simulink model "IMU_Simulation_FxdPts"  (Simulink 7.9)
settings: Solver=FixedStepDiscrete  StartTime=0.0  StopTime=25  FixedStep=.001  RelTol=1e-3
PreLoadFcn:
  | Script_Kalman
values from neighbouring files (symbols this model uses):
  Az = [1 -Ts ;0 1]    [Script_Kalman.m]
  Kz = 1e-3*[.4 ; -.04]    [Script_Kalman.m]
  Ts = .001    (= 0.001)    [Script_Kalman.m]
undefined symbols (not defined in the file or in its folder): DiscIntNeverNeededParam
libraries: simulink x24
settings Model: Creator=Lubin  LastModifiedBy=denis.pretre
settings OptimizationCC: InitFltsAndDblsToZero=on
settings DebuggingCC: MultiTaskCondExecSysMsg=warning  MultiTaskRateTransMsg=warning  FcnCallInpInsideContextMsg=Use local settings  StrictBusMsg=Warning
settings HardwareCC: TargetHWDeviceType=32-bit Generic
settings GRTTargetCC: TargetFcnLib=ansi_tfl_tmw.mat  CombineOutputUpdateFcns=off  GRTInterface=on

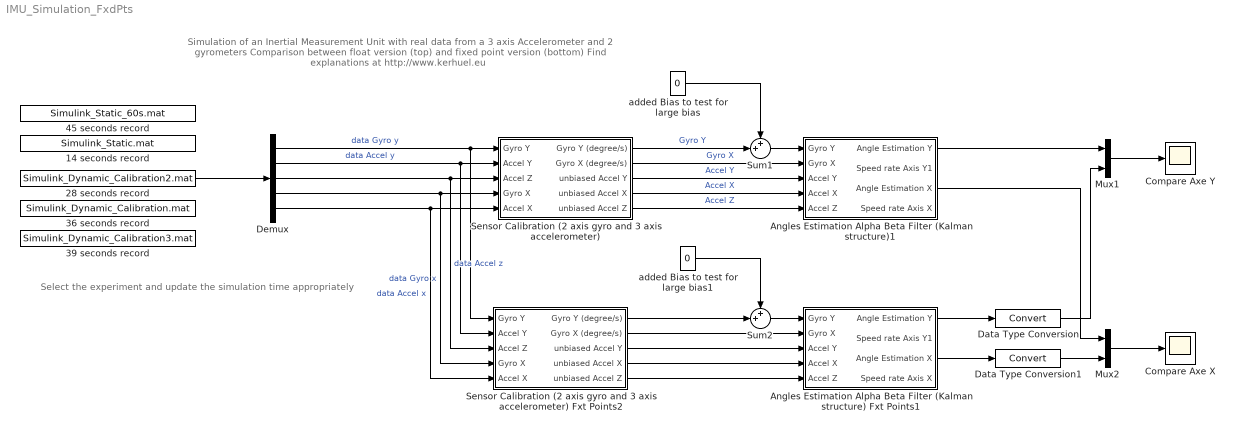
== system IMU_Simulation_FxdPts ==
  note: Simulation of an Inertial Measurement Unit with real data from a 3 axis Accelerometer and 2 gyrometers
      | Comparison between float version (top) and fixed point version (bottom)
      | Find explanations at http://www.kerhuel.eu
  note: Select the experiment and
      | update the simulation time appropriately
  14 seconds record : FromFile  FileName=Simulink_Static.mat  SampleTime=.001
  28 seconds record : FromFile  FileName=Simulink_Dynamic_Calibration2.mat  SampleTime=.001
  36 seconds record : FromFile  FileName=Simulink_Dynamic_Calibration.mat  SampleTime=.001
  39 seconds record : FromFile  FileName=Simulink_Dynamic_Calibration3.mat  SampleTime=.001
  45 seconds record : FromFile  FileName=Simulink_Static_60s.mat  SampleTime=.001
  Angles Estimation Alpha Beta Filter (Kalman structure) Fxt Points1 : Subsystem
  Angles Estimation Alpha Beta Filter (Kalman structure)1 : Subsystem
  Compare Axe X : Scope
      settings: TickLabels=on  TimeRange=25  YMin=-10  YMax=120  SaveName=ScopeData2  Decimation=10
  Compare Axe Y : Scope
      settings: TickLabels=on  TimeRange=25  YMin=0.4  YMax=1.25  SaveName=ScopeData4  Decimation=10
  Data Type Conversion : DataTypeConversion
  Data Type Conversion1 : DataTypeConversion
  Demux : Demux  Outputs=5
  Mux1 : Mux  Inputs=2
  Mux2 : Mux  Inputs=2
  Sensor Calibration (2 axis gyro and 3 axis accelerometer) : Subsystem
  Sensor Calibration (2 axis gyro and 3 axis accelerometer) Fxt Points2 : Subsystem
  Sum1 : Sum  Inputs=++|
  Sum2 : Sum  Inputs=++|
  added Bias to test for large bias : Constant  Value=0
  added Bias to test for large bias1 : Constant  Value=0  OutDataTypeStr=Inherit: Inherit via back propagation
  wires:
  Demux/2 -> Sensor Calibration (2 axis gyro and 3 axis accelerometer)/2(Accel Y), Sensor Calibration (2 axis gyro and 3 axis accelerometer) Fxt Points2/2(Accel Y)  "data Accel y"
  Demux/3 -> Sensor Calibration (2 axis gyro and 3 axis accelerometer)/3(Accel Z), Sensor Calibration (2 axis gyro and 3 axis accelerometer) Fxt Points2/3(Accel Z)  "data Accel z"
  Demux/4 -> Sensor Calibration (2 axis gyro and 3 axis accelerometer)/4(Gyro X), Sensor Calibration (2 axis gyro and 3 axis accelerometer) Fxt Points2/4(Gyro X)  "data Gyro x"
  Demux/5 -> Sensor Calibration (2 axis gyro and 3 axis accelerometer)/5(Accel X), Sensor Calibration (2 axis gyro and 3 axis accelerometer) Fxt Points2/5(Accel X)  "data Accel x"
  Demux/1 -> Sensor Calibration (2 axis gyro and 3 axis accelerometer)/1(Gyro Y), Sensor Calibration (2 axis gyro and 3 axis accelerometer) Fxt Points2/1(Gyro Y)  "data Gyro y"
  Sensor Calibration (2 axis gyro and 3 axis accelerometer)/1(Gyro Y (degree/s)) -> Sum1/2  "Gyro Y"
  Sensor Calibration (2 axis gyro and 3 axis accelerometer)/2(Gyro X (degree/s)) -> Angles Estimation Alpha Beta Filter (Kalman structure)1/2(Gyro X)  "Gyro X"
  Sensor Calibration (2 axis gyro and 3 axis accelerometer)/3(unbiased Accel Y) -> Angles Estimation Alpha Beta Filter (Kalman structure)1/3(Accel Y)  "Accel Y"
  Sensor Calibration (2 axis gyro and 3 axis accelerometer)/4(unbiased Accel X) -> Angles Estimation Alpha Beta Filter (Kalman structure)1/4(Accel X)  "Accel X"
  Sensor Calibration (2 axis gyro and 3 axis accelerometer)/5(unbiased Accel Z) -> Angles Estimation Alpha Beta Filter (Kalman structure)1/5(Accel Z)  "Accel Z"
  Sum1/1 -> Angles Estimation Alpha Beta Filter (Kalman structure)1/1(Gyro Y)
  Mux1/1 -> Compare Axe Y/1
  Sensor Calibration (2 axis gyro and 3 axis accelerometer) Fxt Points2/2(Gyro X (degree/s)) -> Angles Estimation Alpha Beta Filter (Kalman structure) Fxt Points1/2(Gyro X)
  Sensor Calibration (2 axis gyro and 3 axis accelerometer) Fxt Points2/4(unbiased Accel X) -> Angles Estimation Alpha Beta Filter (Kalman structure) Fxt Points1/4(Accel X)
  Sensor Calibration (2 axis gyro and 3 axis accelerometer) Fxt Points2/5(unbiased Accel Z) -> Angles Estimation Alpha Beta Filter (Kalman structure) Fxt Points1/5(Accel Z)
  Angles Estimation Alpha Beta Filter (Kalman structure)1/1(Angle Estimation Y) -> Mux1/1
  Angles Estimation Alpha Beta Filter (Kalman structure) Fxt Points1/1(Angle Estimation Y) -> Data Type Conversion/1
  Data Type Conversion/1 -> Mux1/2
  added Bias to test for large bias/1 -> Sum1/1
  Mux2/1 -> Compare Axe X/1
  Angles Estimation Alpha Beta Filter (Kalman structure) Fxt Points1/3(Angle Estimation X) -> Data Type Conversion1/1
  Data Type Conversion1/1 -> Mux2/2
  Angles Estimation Alpha Beta Filter (Kalman structure)1/3(Angle Estimation X) -> Mux2/1
  Sensor Calibration (2 axis gyro and 3 axis accelerometer) Fxt Points2/3(unbiased Accel Y) -> Angles Estimation Alpha Beta Filter (Kalman structure) Fxt Points1/3(Accel Y)
  28 seconds record/1 -> Demux/1
  added Bias to test for large bias1/1 -> Sum2/1
  Sensor Calibration (2 axis gyro and 3 axis accelerometer) Fxt Points2/1(Gyro Y (degree/s)) -> Sum2/2
  Sum2/1 -> Angles Estimation Alpha Beta Filter (Kalman structure) Fxt Points1/1(Gyro Y)

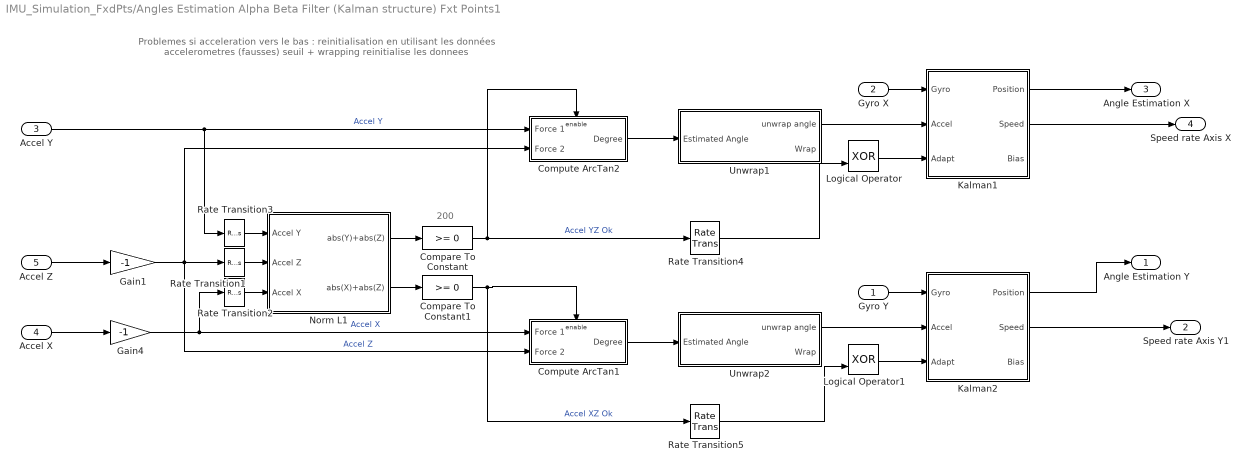
== system IMU_Simulation_FxdPts/Angles Estimation Alpha Beta Filter (Kalman structure) Fxt Points1 ==
  note: 200
  note: Problemes si acceleration vers le bas : reinitialisation en utilisant les données accelerometres (fausses)
      | seuil + wrapping reinitialise les donnees
  Gyro Y : Inport
  Gyro X : Inport  Port=2
  Accel Y : Inport  Port=3
  Accel X : Inport  Port=4
  Accel Z : Inport  Port=5
  Compare To Constant : simulink/Logic and Bit Operations/Compare To Constant  relop=>=  const=0  OutDataTypeStr=boolean  ZeroCross=off
  Compare To Constant1 : simulink/Logic and Bit Operations/Compare To Constant  relop=>=  const=0  OutDataTypeStr=boolean  ZeroCross=off
  Compute ArcTan1 : Subsystem
  Compute ArcTan2 : Subsystem
  Gain1 : Gain  Gain=-1  OutDataTypeStr=Inherit: Same as input
  Gain4 : Gain  Gain=-1  OutDataTypeStr=Inherit: Same as input
  Kalman1 : Subsystem
  Kalman2 : Subsystem
  Logical Operator : Logic  Operator=XOR  AllPortsSameDT=off  OutDataTypeStr=boolean
  Logical Operator1 : Logic  Operator=XOR  AllPortsSameDT=off  OutDataTypeStr=boolean
  Norm L1 : Subsystem
  Rate Transition1 : RateTransition  Integrity=off  OutPortSampleTime=.2
  Rate Transition2 : RateTransition  Integrity=off  OutPortSampleTime=.2
  Rate Transition3 : RateTransition  Integrity=off  OutPortSampleTime=.2
  Rate Transition4 : RateTransition  Integrity=off  OutPortSampleTime=.001
  Rate Transition5 : RateTransition  Integrity=off  OutPortSampleTime=.001
  Unwrap1 : Subsystem
  Unwrap2 : Subsystem
  Angle Estimation Y : Outport
  Speed rate Axis Y1 : Outport  Port=2
  Angle Estimation X : Outport  Port=3
  Speed rate Axis X : Outport  Port=4
  wires:
  Kalman2/2(Speed) -> Speed rate Axis Y1/1
  Kalman1/2(Speed) -> Speed rate Axis X/1
  Unwrap2/1(unwrap angle) -> Kalman2/2(Accel)
  Logical Operator/1 -> Kalman1/3(Adapt)
  Rate Transition5/1 -> Logical Operator1/2
  Gain1/1 -> Compute ArcTan1/2(Force 2), Compute ArcTan2/2(Force 2), Rate Transition1/1  "Accel Z"
  Logical Operator1/1 -> Kalman2/3(Adapt)
  Rate Transition4/1 -> Logical Operator/2
  Unwrap1/1(unwrap angle) -> Kalman1/2(Accel)
  Rate Transition3/1 -> Norm L1/1(Accel Y)
  Rate Transition2/1 -> Norm L1/3(Accel X)
  Rate Transition1/1 -> Norm L1/2(Accel Z)
  Kalman2/1(Position) -> Angle Estimation Y/1
  Kalman1/1(Position) -> Angle Estimation X/1
  Compare To Constant1/1 -> Compute ArcTan1/Enable, Rate Transition5/1  "Accel XZ Ok"
  Compare To Constant/1 -> Compute ArcTan2/Enable, Rate Transition4/1  "Accel YZ Ok"
  Norm L1/1(abs(Y)+abs(Z)) -> Compare To Constant/1
  Norm L1/2(abs(X)+abs(Z)) -> Compare To Constant1/1
  Accel Z/1 -> Gain1/1
  Gain4/1 -> Compute ArcTan1/1(Force 1), Rate Transition2/1  "Accel X"
  Compute ArcTan2/1(Degree) -> Unwrap1/1(Estimated Angle)
  Compute ArcTan1/1(Degree) -> Unwrap2/1(Estimated Angle)
  Accel X/1 -> Gain4/1
  Accel Y/1 -> Rate Transition3/1, Compute ArcTan2/1(Force 1)  "Accel Y"
  Gyro X/1 -> Kalman1/1(Gyro)
  Gyro Y/1 -> Kalman2/1(Gyro)

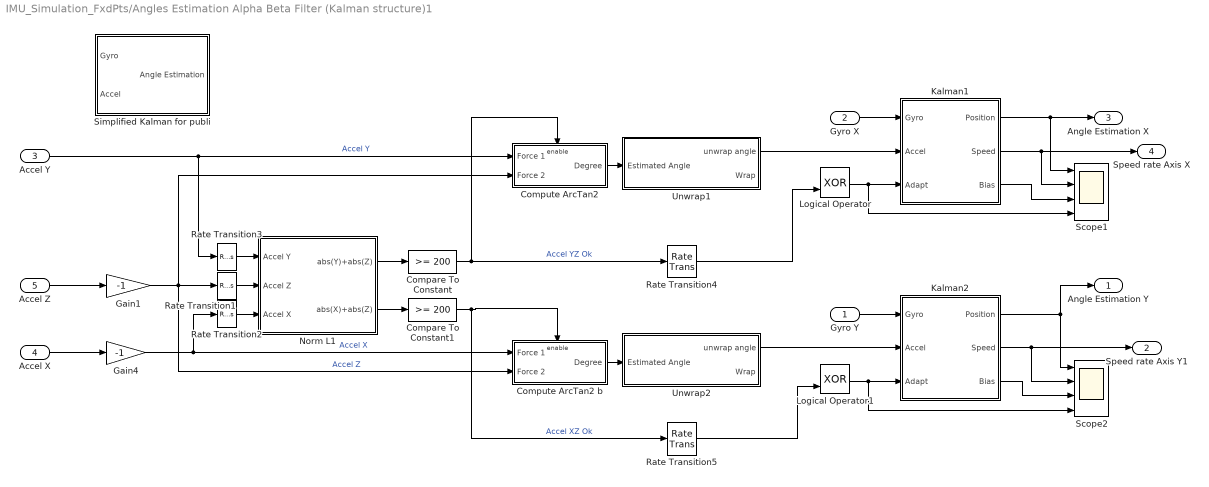
== system IMU_Simulation_FxdPts/Angles Estimation Alpha Beta Filter (Kalman structure)1 ==
  Gyro Y : Inport
  Gyro X : Inport  Port=2
  Accel Y : Inport  Port=3
  Accel X : Inport  Port=4
  Accel Z : Inport  Port=5
  Compare To Constant : simulink/Logic and Bit Operations/Compare To Constant  relop=>=  const=200  OutDataTypeStr=boolean  ZeroCross=off
  Compare To Constant1 : simulink/Logic and Bit Operations/Compare To Constant  relop=>=  const=200  OutDataTypeStr=boolean  ZeroCross=off
  Compute ArcTan2 : Subsystem
  Compute ArcTan2 b : Subsystem
  Gain1 : Gain  Gain=-1
  Gain4 : Gain  Gain=-1
  Kalman1 : Subsystem
  Kalman2 : Subsystem
  Logical Operator : Logic  Operator=XOR  AllPortsSameDT=off  OutDataTypeStr=boolean
  Logical Operator1 : Logic  Operator=XOR  AllPortsSameDT=off  OutDataTypeStr=boolean
  Norm L1 : Subsystem
  Rate Transition1 : RateTransition  Integrity=off  OutPortSampleTime=.2
  Rate Transition2 : RateTransition  Integrity=off  OutPortSampleTime=.2
  Rate Transition3 : RateTransition  Integrity=off  OutPortSampleTime=.2
  Rate Transition4 : RateTransition  Integrity=off  OutPortSampleTime=.001
  Rate Transition5 : RateTransition  Integrity=off  OutPortSampleTime=.001
  Scope1 : Scope  NumInputPorts=4
      settings: TimeRange=9.424342105263159  YMin=-375~-20~-27.5~0  YMax=-150~40~2.5~1
  Scope2 : Scope  NumInputPorts=4
      settings: TimeRange=9.424342105263159  YMin=-375~-20~-27.5~0  YMax=-150~40~2.5~1
  Simplified Kalman for publi : Subsystem
  Unwrap1 : Subsystem
  Unwrap2 : Subsystem
  Angle Estimation Y : Outport
  Speed rate Axis Y1 : Outport  Port=2
  Angle Estimation X : Outport  Port=3
  Speed rate Axis X : Outport  Port=4
  wires:
  Kalman1/3(Bias) -> Scope1/3
  Kalman2/3(Bias) -> Scope2/3
  Kalman2/2(Speed) -> Speed rate Axis Y1/1, Scope2/2
  Kalman1/2(Speed) -> Speed rate Axis X/1, Scope1/2
  Unwrap2/1(unwrap angle) -> Kalman2/2(Accel)
  Logical Operator/1 -> Scope1/4, Kalman1/3(Adapt)
  Rate Transition5/1 -> Logical Operator1/2
  Gain1/1 -> Rate Transition1/1, Compute ArcTan2/2(Force 2), Compute ArcTan2 b/2(Force 2)  "Accel Z"
  Logical Operator1/1 -> Kalman2/3(Adapt), Scope2/4
  Rate Transition4/1 -> Logical Operator/2
  Unwrap1/1(unwrap angle) -> Kalman1/2(Accel)
  Rate Transition3/1 -> Norm L1/1(Accel Y)
  Rate Transition2/1 -> Norm L1/3(Accel X)
  Rate Transition1/1 -> Norm L1/2(Accel Z)
  Kalman2/1(Position) -> Scope2/1, Angle Estimation Y/1
  Kalman1/1(Position) -> Scope1/1, Angle Estimation X/1
  Compare To Constant1/1 -> Rate Transition5/1, Compute ArcTan2 b/Enable  "Accel XZ Ok"
  Compare To Constant/1 -> Rate Transition4/1, Compute ArcTan2/Enable  "Accel YZ Ok"
  Norm L1/1(abs(Y)+abs(Z)) -> Compare To Constant/1
  Norm L1/2(abs(X)+abs(Z)) -> Compare To Constant1/1
  Accel Z/1 -> Gain1/1
  Gain4/1 -> Rate Transition2/1, Compute ArcTan2 b/1(Force 1)  "Accel X"
  Compute ArcTan2/1(Degree) -> Unwrap1/1(Estimated Angle)
  Compute ArcTan2 b/1(Degree) -> Unwrap2/1(Estimated Angle)
  Accel X/1 -> Gain4/1
  Accel Y/1 -> Compute ArcTan2/1(Force 1), Rate Transition3/1  "Accel Y"
  Gyro X/1 -> Kalman1/1(Gyro)
  Gyro Y/1 -> Kalman2/1(Gyro)

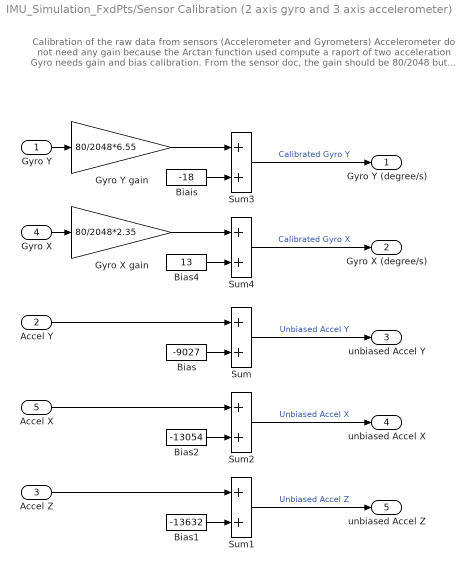
== system IMU_Simulation_FxdPts/Sensor Calibration (2 axis gyro and 3 axis accelerometer) ==
  note: Calibration of the raw data from sensors (Accelerometer and Gyrometers)
      | Accelerometer do not need any gain because the Arctan function used compute a raport of two acceleration
      | Gyro needs gain and bias calibration. From the sensor doc, the gain should be 80/2048 but...
  Gyro Y : Inport
  Accel Y : Inport  Port=2
  Accel Z : Inport  Port=3
  Gyro X : Inport  Port=4
  Accel X : Inport  Port=5
  "Biais " : Constant  Value=-18
  Bias : Constant  Value=-9027
  Bias1 : Constant  Value=-13632
  Bias2 : Constant  Value=-13054
  Bias4 : Constant  Value=13
  Gyro X gain : Gain  Gain=80/2048*2.35  OutDataTypeStr=float('double')
  Gyro Y gain : Gain  Gain=80/2048*6.55  OutDataTypeStr=float('double')
  Sum{,1..4} (5 alike) : Sum
  Gyro Y (degree/s) : Outport
  Gyro X (degree/s) : Outport  Port=2
  unbiased Accel Y : Outport  Port=3
  unbiased Accel X : Outport  Port=4
  unbiased Accel Z : Outport  Port=5
  wires:
  Bias/1 -> Sum/2
  Bias1/1 -> Sum1/2
  Bias2/1 -> Sum2/2
  Gyro Y/1 -> Gyro Y gain/1
  Accel Y/1 -> Sum/1
  Sum/1 -> unbiased Accel Y/1  "Unbiased Accel Y"
  Accel Z/1 -> Sum1/1
  Sum1/1 -> unbiased Accel Z/1  "Unbiased Accel Z"
  Gyro X/1 -> Gyro X gain/1
  Accel X/1 -> Sum2/1
  Sum2/1 -> unbiased Accel X/1  "Unbiased Accel X"
  Gyro Y gain/1 -> Sum3/1
  Sum3/1 -> Gyro Y (degree/s)/1  "Calibrated Gyro Y"
  "Biais "/1 -> Sum3/2
  Gyro X gain/1 -> Sum4/1
  Sum4/1 -> Gyro X (degree/s)/1  "Calibrated Gyro X"
  Bias4/1 -> Sum4/2

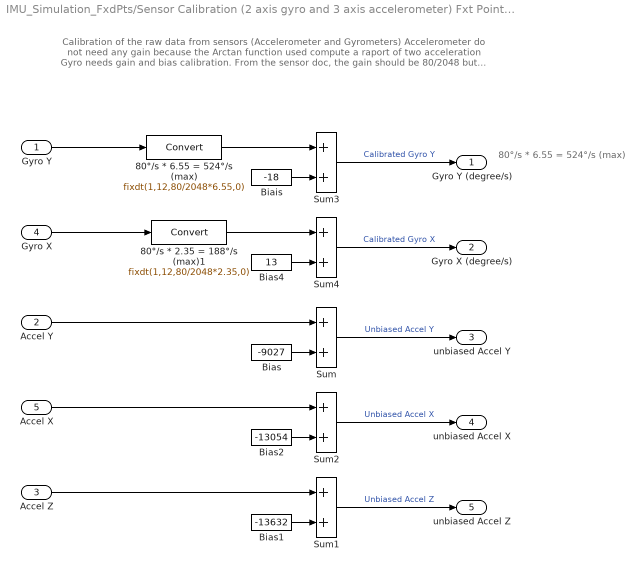
== system IMU_Simulation_FxdPts/Sensor Calibration (2 axis gyro and 3 axis accelerometer) Fxt Points2 ==
  note: Calibration of the raw data from sensors (Accelerometer and Gyrometers)
      | Accelerometer do not need any gain because the Arctan function used compute a raport of two acceleration
      | Gyro needs gain and bias calibration. From the sensor doc, the gain should be 80/2048 but...
  note: 80°/s * 6.55 = 524°/s (max)
  Gyro Y : Inport
  Accel Y : Inport  Port=2
  Accel Z : Inport  Port=3
  Gyro X : Inport  Port=4
  Accel X : Inport  Port=5
  80°/s * 2.35 = 188°/s (max)1 : DataTypeConversion  OutDataTypeStr=fixdt(1,12,80/2048*2.35,0)  ConvertRealWorld=Stored Integer (SI)
  80°/s * 6.55 = 524°/s (max) : DataTypeConversion  OutDataTypeStr=fixdt(1,12,80/2048*6.55,0)  ConvertRealWorld=Stored Integer (SI)
  "Biais " : Constant  Value=-18  OutDataTypeStr=Inherit: Inherit via back propagation
  Bias : Constant  Value=-9027  OutDataTypeStr=Inherit: Inherit via back propagation
  Bias1 : Constant  Value=-13632  OutDataTypeStr=Inherit: Inherit via back propagation
  Bias2 : Constant  Value=-13054  OutDataTypeStr=Inherit: Inherit via back propagation
  Bias4 : Constant  Value=13  OutDataTypeStr=Inherit: Inherit via back propagation
  Sum : Sum  OutDataTypeStr=int16
  Sum1 : Sum  OutDataTypeStr=int16
  Sum2 : Sum  OutDataTypeStr=int16
  Sum3 : Sum
  Sum4 : Sum
  Gyro Y (degree/s) : Outport
  Gyro X (degree/s) : Outport  Port=2
  unbiased Accel Y : Outport  Port=3
  unbiased Accel X : Outport  Port=4
  unbiased Accel Z : Outport  Port=5
  wires:
  Bias4/1 -> Sum4/2
  Sum4/1 -> Gyro X (degree/s)/1  "Calibrated Gyro X"
  80°/s * 2.35 = 188°/s (max)1/1 -> Sum4/1
  "Biais "/1 -> Sum3/2
  Sum3/1 -> Gyro Y (degree/s)/1  "Calibrated Gyro Y"
  80°/s * 6.55 = 524°/s (max)/1 -> Sum3/1
  Sum2/1 -> unbiased Accel X/1  "Unbiased Accel X"
  Accel X/1 -> Sum2/1
  Gyro X/1 -> 80°/s * 2.35 = 188°/s (max)1/1
  Sum1/1 -> unbiased Accel Z/1  "Unbiased Accel Z"
  Accel Z/1 -> Sum1/1
  Sum/1 -> unbiased Accel Y/1  "Unbiased Accel Y"
  Accel Y/1 -> Sum/1
  Gyro Y/1 -> 80°/s * 6.55 = 524°/s (max)/1
  Bias2/1 -> Sum2/2
  Bias1/1 -> Sum1/2
  Bias/1 -> Sum/2

== system IMU_Simulation_FxdPts/Angles Estimation Alpha Beta Filter (Kalman structure) Fxt Points1/Compute ArcTan1 ==
  Force 1 : Inport
  Force 2 : Inport  Port=2
  Enable : EnablePort  StatesWhenEnabling=reset
  180/pi : DataTypeConversion  OutDataTypeStr=fixdt(1,16,180/pi*2^-12,0)  ConvertRealWorld=Stored Integer (SI)
  80°/s * 6.55 = 524°/s (max) : DataTypeConversion  OutDataTypeStr=single
  80°/s * 6.55 = 524°/s (max)1 : DataTypeConversion  OutDataTypeStr=single
  80°/s * 6.55 = 524°/s (max)2 : DataTypeConversion  OutDataTypeStr=fixdt(1,16,12)
  Trigonometric Function1 : Trigonometry  Operator=atan2  OutputSignalType=real
  Degree : Outport
  wires:
  Trigonometric Function1/1 -> 80°/s * 6.55 = 524°/s (max)2/1
  180/pi/1 -> Degree/1
  Force 1/1 -> 80°/s * 6.55 = 524°/s (max)/1
  Force 2/1 -> 80°/s * 6.55 = 524°/s (max)1/1
  80°/s * 6.55 = 524°/s (max)/1 -> Trigonometric Function1/1
  80°/s * 6.55 = 524°/s (max)1/1 -> Trigonometric Function1/2
  80°/s * 6.55 = 524°/s (max)2/1 -> 180/pi/1

== system IMU_Simulation_FxdPts/Angles Estimation Alpha Beta Filter (Kalman structure) Fxt Points1/Compute ArcTan2 ==
  Force 1 : Inport
  Force 2 : Inport  Port=2
  Enable : EnablePort  StatesWhenEnabling=reset
  180/pi : DataTypeConversion  OutDataTypeStr=fixdt(1,16,180/pi*2^-12,0)  ConvertRealWorld=Stored Integer (SI)
  80°/s * 6.55 = 524°/s (max) : DataTypeConversion  OutDataTypeStr=single
  80°/s * 6.55 = 524°/s (max)1 : DataTypeConversion  OutDataTypeStr=single
  80°/s * 6.55 = 524°/s (max)2 : DataTypeConversion  OutDataTypeStr=fixdt(1,16,12)
  Trigonometric Function1 : Trigonometry  Operator=atan2  OutputSignalType=real
  Degree : Outport
  wires:
  80°/s * 6.55 = 524°/s (max)2/1 -> 180/pi/1
  80°/s * 6.55 = 524°/s (max)1/1 -> Trigonometric Function1/2
  80°/s * 6.55 = 524°/s (max)/1 -> Trigonometric Function1/1
  Force 2/1 -> 80°/s * 6.55 = 524°/s (max)1/1
  Force 1/1 -> 80°/s * 6.55 = 524°/s (max)/1
  180/pi/1 -> Degree/1
  Trigonometric Function1/1 -> 80°/s * 6.55 = 524°/s (max)2/1

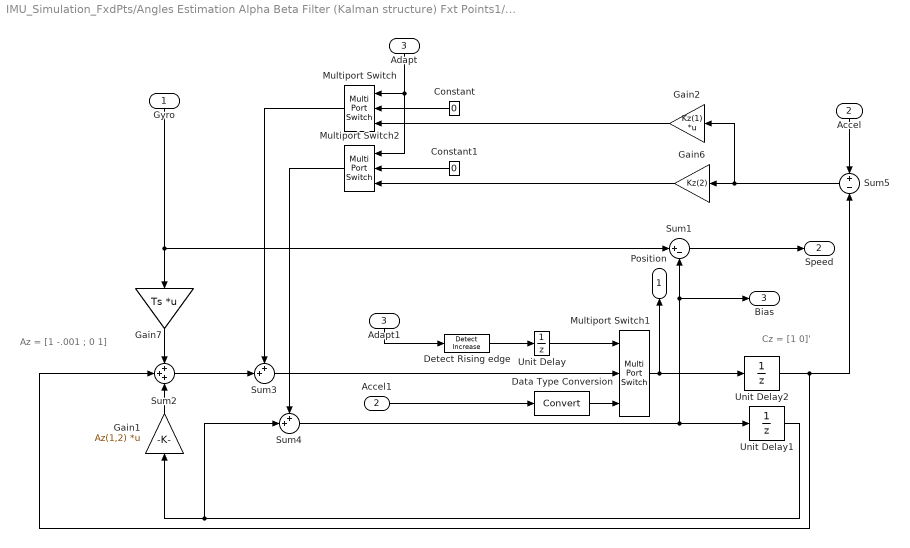
== system IMU_Simulation_FxdPts/Angles Estimation Alpha Beta Filter (Kalman structure) Fxt Points1/Kalman1 ==
  note: Az = [1 -.001 ; 0 1]
  note: Cz = [1 0]'
  Gyro : Inport
  Accel : Inport  Port=2
  Adapt : Inport  Port=3
  Accel1 : InportShadow  Port=2
  Adapt1 : InportShadow  Port=3
  Constant : Constant  Value=0  OutDataTypeStr=Inherit: Inherit via back propagation
  Constant1 : Constant  Value=0  OutDataTypeStr=Inherit: Inherit via back propagation
  Data Type Conversion : DataTypeConversion
  Detect Rising edge : simulink/Logic and Bit Operations/Detect Increase  vinit=0  InputProcessing=Inherited  OutDataTypeStr=uint8
  Gain1 : Gain  Gain=Az(1,2)  Multiplication=Matrix(K*u)  OutDataTypeStr=fixdt(1,32,36)
  Gain2 : Gain  Gain=Kz(1)  Multiplication=Matrix(K*u)  ParamDataTypeStr=fixdt(1,32,42)  OutDataTypeStr=fixdt(1,16,20)  SaturateOnIntegerOverflow=on
  Gain6 : Gain  Gain=Kz(2)  ParamDataTypeStr=fixdt(1,32,45)  OutDataTypeStr=fixdt(1,16,23)  SaturateOnIntegerOverflow=on
  Gain7 : Gain  Gain=Ts  Multiplication=Matrix(K*u)  OutDataTypeStr=Inherit: Inherit via back propagation
  Multiport Switch : MultiPortSwitch  DataPortOrder=Zero-based contiguous  Inputs=2  zeroidx=on
  Multiport Switch1 : MultiPortSwitch  DataPortOrder=Zero-based contiguous  Inputs=2  zeroidx=on  OutDataTypeStr=Inherit: Inherit via back propagation
  Multiport Switch2 : MultiPortSwitch  DataPortOrder=Zero-based contiguous  Inputs=2  zeroidx=on
  Sum1 : Sum  Inputs=|+-  OutDataTypeStr=Inherit: Same as first input
  Sum2 : Sum  Inputs=+++  OutDataTypeStr=fixdt(1,32,22)
  Sum3 : Sum  Inputs=++|  OutDataTypeStr=fixdt(1,32,22)
  Sum4 : Sum  Inputs=++|  OutDataTypeStr=fixdt(1,32,26)
  Sum5 : Sum  Inputs=+-  OutDataTypeStr=fixdt(1,16,9)  SaturateOnIntegerOverflow=on
  Unit Delay : UnitDelay  SampleTime=-1
  Unit Delay1 : UnitDelay  SampleTime=-1
  Unit Delay2 : UnitDelay  SampleTime=-1
  Position : Outport  OutDataTypeStr=fixdt(1,32,22)
  Speed : Outport  Port=2
  Bias : Outport  Port=3
  wires:
  Gyro/1 -> Sum1/1, Gain7/1
  Gain6/1 -> Multiport Switch2/3
  Unit Delay1/1 -> Sum4/2, Gain1/1
  Multiport Switch1/1 -> Position/1, Unit Delay2/1
  Sum4/1 -> Bias/1, Sum1/2, Unit Delay1/1
  Data Type Conversion/1 -> Multiport Switch1/3
  Accel1/1 -> Data Type Conversion/1
  Sum3/1 -> Multiport Switch1/2
  Multiport Switch2/1 -> Sum4/1
  Multiport Switch/1 -> Sum3/1
  Constant1/1 -> Multiport Switch2/2
  Gain2/1 -> Multiport Switch/3
  Gain1/1 -> Sum2/3
  Sum1/1 -> Speed/1
  Unit Delay/1 -> Multiport Switch1/1
  Accel/1 -> Sum5/1
  Gain7/1 -> Sum2/1
  Sum5/1 -> Gain2/1, Gain6/1
  Sum2/1 -> Sum3/2
  Unit Delay2/1 -> Sum2/2, Sum5/2
  Adapt/1 -> Multiport Switch2/1, Multiport Switch/1
  Constant/1 -> Multiport Switch/2
  Detect Rising edge/1 -> Unit Delay/1
  Adapt1/1 -> Detect Rising edge/1

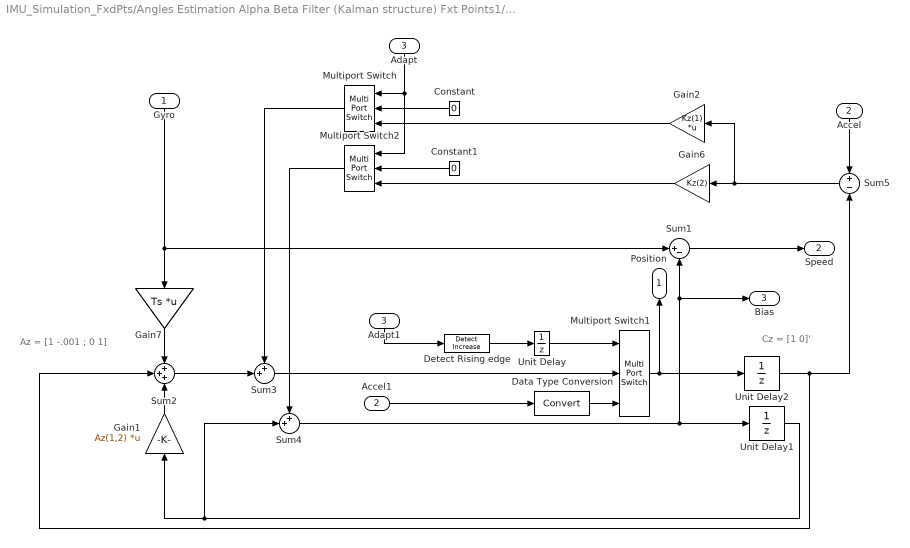
== system IMU_Simulation_FxdPts/Angles Estimation Alpha Beta Filter (Kalman structure) Fxt Points1/Kalman2 ==
  note: Cz = [1 0]'
  note: Az = [1 -.001 ; 0 1]
  Gyro : Inport
  Accel : Inport  Port=2
  Adapt : Inport  Port=3
  Accel1 : InportShadow  Port=2
  Adapt1 : InportShadow  Port=3
  Constant : Constant  Value=0  OutDataTypeStr=Inherit: Inherit via back propagation
  Constant1 : Constant  Value=0  OutDataTypeStr=Inherit: Inherit via back propagation
  Data Type Conversion : DataTypeConversion
  Detect Rising edge : simulink/Logic and Bit Operations/Detect Increase  vinit=0  InputProcessing=Inherited  OutDataTypeStr=uint8
  Gain1 : Gain  Gain=Az(1,2)  Multiplication=Matrix(K*u)  OutDataTypeStr=fixdt(1,32,36)
  Gain2 : Gain  Gain=Kz(1)  Multiplication=Matrix(K*u)  ParamDataTypeStr=fixdt(1,32,42)  OutDataTypeStr=fixdt(1,16,20)  SaturateOnIntegerOverflow=on
  Gain6 : Gain  Gain=Kz(2)  ParamDataTypeStr=fixdt(1,32,45)  OutDataTypeStr=fixdt(1,16,23)  SaturateOnIntegerOverflow=on
  Gain7 : Gain  Gain=Ts  Multiplication=Matrix(K*u)  OutDataTypeStr=Inherit: Inherit via back propagation
  Multiport Switch : MultiPortSwitch  DataPortOrder=Zero-based contiguous  Inputs=2  zeroidx=on
  Multiport Switch1 : MultiPortSwitch  DataPortOrder=Zero-based contiguous  Inputs=2  zeroidx=on  OutDataTypeStr=Inherit: Inherit via back propagation
  Multiport Switch2 : MultiPortSwitch  DataPortOrder=Zero-based contiguous  Inputs=2  zeroidx=on
  Sum1 : Sum  Inputs=|+-  OutDataTypeStr=Inherit: Same as first input
  Sum2 : Sum  Inputs=+++  OutDataTypeStr=fixdt(1,32,22)
  Sum3 : Sum  Inputs=++|  OutDataTypeStr=fixdt(1,32,22)
  Sum4 : Sum  Inputs=++|  OutDataTypeStr=fixdt(1,32,26)
  Sum5 : Sum  Inputs=+-  OutDataTypeStr=fixdt(1,16,9)  SaturateOnIntegerOverflow=on
  Unit Delay : UnitDelay  SampleTime=-1
  Unit Delay1 : UnitDelay  SampleTime=-1
  Unit Delay2 : UnitDelay  SampleTime=-1
  Position : Outport  OutDataTypeStr=fixdt(1,32,22)
  Speed : Outport  Port=2
  Bias : Outport  Port=3
  wires:
  Adapt1/1 -> Detect Rising edge/1
  Detect Rising edge/1 -> Unit Delay/1
  Constant/1 -> Multiport Switch/2
  Adapt/1 -> Multiport Switch/1, Multiport Switch2/1
  Unit Delay2/1 -> Sum5/2, Sum2/2
  Sum2/1 -> Sum3/2
  Sum5/1 -> Gain6/1, Gain2/1
  Gain7/1 -> Sum2/1
  Accel/1 -> Sum5/1
  Unit Delay/1 -> Multiport Switch1/1
  Sum1/1 -> Speed/1
  Gain1/1 -> Sum2/3
  Gain2/1 -> Multiport Switch/3
  Constant1/1 -> Multiport Switch2/2
  Multiport Switch/1 -> Sum3/1
  Multiport Switch2/1 -> Sum4/1
  Sum3/1 -> Multiport Switch1/2
  Accel1/1 -> Data Type Conversion/1
  Data Type Conversion/1 -> Multiport Switch1/3
  Sum4/1 -> Unit Delay1/1, Sum1/2, Bias/1
  Multiport Switch1/1 -> Unit Delay2/1, Position/1
  Unit Delay1/1 -> Gain1/1, Sum4/2
  Gain6/1 -> Multiport Switch2/3
  Gyro/1 -> Gain7/1, Sum1/1

== system IMU_Simulation_FxdPts/Angles Estimation Alpha Beta Filter (Kalman structure) Fxt Points1/Norm L1 ==
  Accel Y : Inport
  Accel Z : Inport  Port=2
  Accel X : Inport  Port=3
  Abs : Abs
  Abs1 : Abs
  Abs2 : Abs
  Sum1 : Sum
  Sum3 : Sum
  abs(Y)+abs(Z) : Outport
  abs(X)+abs(Z) : Outport  Port=2
  wires:
  Sum1/1 -> abs(X)+abs(Z)/1
  Accel X/1 -> Abs2/1
  Abs2/1 -> Sum1/2
  Sum3/1 -> abs(Y)+abs(Z)/1
  Accel Z/1 -> Abs1/1
  Accel Y/1 -> Abs/1
  Abs1/1 -> Sum3/2, Sum1/1
  Abs/1 -> Sum3/1

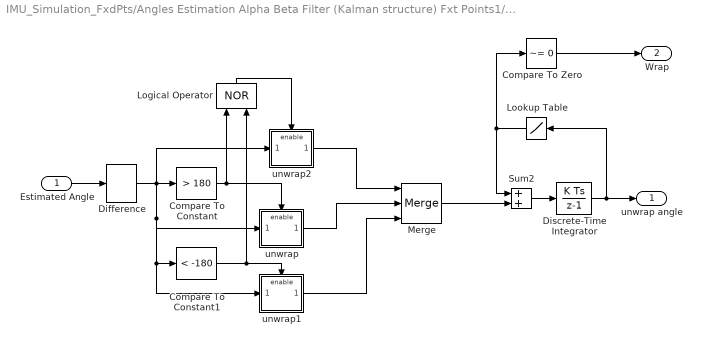
== system IMU_Simulation_FxdPts/Angles Estimation Alpha Beta Filter (Kalman structure) Fxt Points1/Unwrap1 ==
  Estimated Angle : Inport
  Compare To Constant : simulink/Logic and Bit Operations/Compare To Constant  relop=>  const=180  OutDataTypeStr=uint8  ZeroCross=off
  Compare To Constant1 : simulink/Logic and Bit Operations/Compare To Constant  relop=<  const=-180  OutDataTypeStr=uint8  ZeroCross=off
  Compare To Zero : simulink/Logic and Bit Operations/Compare To Zero  relop=~=  OutDataTypeStr=uint8  ZeroCross=off
  Difference : simulink/Discrete/Difference  ICPrevInput=0.0  InputProcessing=Inherited  OutMin=[]  OutMax=[]  OutDataType=sfix(16)  OutScaling=2^-10  DoSatur=off
  Discrete-Time Integrator : DiscreteIntegrator  gainval=1000  SampleTime=-1  ICPrevOutput=DiscIntNeverNeededParam  ICPrevScaledInput=DiscIntNeverNeededParam
  Logical Operator : Logic  Operator=NOR  AllPortsSameDT=off  OutDataTypeStr=boolean
  Lookup Table : Lookup  InputValues=[-450 -195 195]  Table=[+360 0 -360]  LookUpMeth=Use Input Below
  Merge : Merge  Inputs=3
  Sum2 : Sum
  unwrap : Subsystem  TreatAsAtomicUnit=on
  unwrap1 : Subsystem  TreatAsAtomicUnit=on
  unwrap2 : Subsystem  TreatAsAtomicUnit=on
  unwrap angle : Outport
  Wrap : Outport  Port=2
  wires:
  Discrete-Time Integrator/1 -> unwrap angle/1, Lookup Table/1
  Estimated Angle/1 -> Difference/1
  unwrap1/1(Out1) -> Merge/3
  unwrap/1(Out1) -> Merge/2
  unwrap2/1(Out1) -> Merge/1
  Logical Operator/1 -> unwrap2/Enable
  Compare To Constant1/1 -> Logical Operator/2, unwrap1/Enable
  Compare To Constant/1 -> unwrap/Enable, Logical Operator/1
  Difference/1 -> unwrap2/1(In1), unwrap1/1(In1), Compare To Constant1/1, unwrap/1(In1), Compare To Constant/1
  Sum2/1 -> Discrete-Time Integrator/1
  Merge/1 -> Sum2/2
  Lookup Table/1 -> Sum2/1, Compare To Zero/1
  Compare To Zero/1 -> Wrap/1

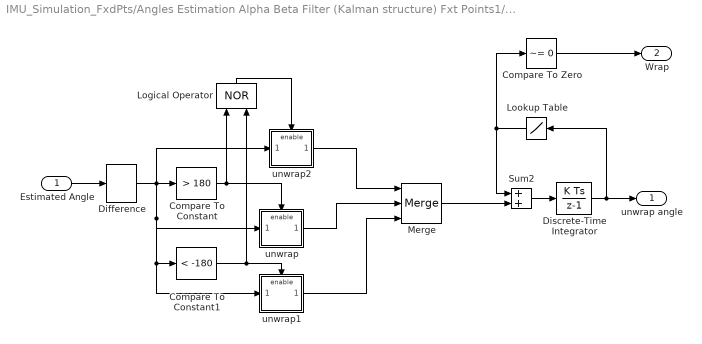
== system IMU_Simulation_FxdPts/Angles Estimation Alpha Beta Filter (Kalman structure) Fxt Points1/Unwrap2 ==
  Estimated Angle : Inport
  Compare To Constant : simulink/Logic and Bit Operations/Compare To Constant  relop=>  const=180  OutDataTypeStr=uint8  ZeroCross=off
  Compare To Constant1 : simulink/Logic and Bit Operations/Compare To Constant  relop=<  const=-180  OutDataTypeStr=uint8  ZeroCross=off
  Compare To Zero : simulink/Logic and Bit Operations/Compare To Zero  relop=~=  OutDataTypeStr=uint8  ZeroCross=off
  Difference : simulink/Discrete/Difference  ICPrevInput=0.0  InputProcessing=Inherited  OutMin=[]  OutMax=[]  OutDataType=sfix(16)  OutScaling=2^-10  DoSatur=off
  Discrete-Time Integrator : DiscreteIntegrator  gainval=1000  SampleTime=-1  ICPrevOutput=DiscIntNeverNeededParam  ICPrevScaledInput=DiscIntNeverNeededParam
  Logical Operator : Logic  Operator=NOR  AllPortsSameDT=off  OutDataTypeStr=boolean
  Lookup Table : Lookup  InputValues=[-450 -195 195]  Table=[+360 0 -360]  LookUpMeth=Use Input Below
  Merge : Merge  Inputs=3
  Sum2 : Sum
  unwrap : Subsystem  TreatAsAtomicUnit=on
  unwrap1 : Subsystem  TreatAsAtomicUnit=on
  unwrap2 : Subsystem  TreatAsAtomicUnit=on
  unwrap angle : Outport
  Wrap : Outport  Port=2
  wires:
  Compare To Zero/1 -> Wrap/1
  Lookup Table/1 -> Compare To Zero/1, Sum2/1
  Merge/1 -> Sum2/2
  Sum2/1 -> Discrete-Time Integrator/1
  Difference/1 -> Compare To Constant/1, unwrap/1(In1), Compare To Constant1/1, unwrap1/1(In1), unwrap2/1(In1)
  Compare To Constant/1 -> Logical Operator/1, unwrap/Enable
  Compare To Constant1/1 -> unwrap1/Enable, Logical Operator/2
  Logical Operator/1 -> unwrap2/Enable
  unwrap2/1(Out1) -> Merge/1
  unwrap/1(Out1) -> Merge/2
  unwrap1/1(Out1) -> Merge/3
  Estimated Angle/1 -> Difference/1
  Discrete-Time Integrator/1 -> Lookup Table/1, unwrap angle/1

== system IMU_Simulation_FxdPts/Angles Estimation Alpha Beta Filter (Kalman structure)1/Compute ArcTan2 ==
  Force 1 : Inport
  Force 2 : Inport  Port=2
  Enable : EnablePort  StatesWhenEnabling=reset
  Gain1 : Gain  Gain=180/pi  OutDataTypeStr=float('double')
  Trigonometric Function1 : Trigonometry  Operator=atan2  OutputSignalType=real
  Degree : Outport
  wires:
  Force 2/1 -> Trigonometric Function1/2
  Force 1/1 -> Trigonometric Function1/1
  Gain1/1 -> Degree/1
  Trigonometric Function1/1 -> Gain1/1

== system IMU_Simulation_FxdPts/Angles Estimation Alpha Beta Filter (Kalman structure)1/Compute ArcTan2 b ==
  Force 1 : Inport
  Force 2 : Inport  Port=2
  Enable : EnablePort  StatesWhenEnabling=reset
  Gain1 : Gain  Gain=180/pi  OutDataTypeStr=float('double')
  Trigonometric Function1 : Trigonometry  Operator=atan2  OutputSignalType=real
  Degree : Outport
  wires:
  Trigonometric Function1/1 -> Gain1/1
  Gain1/1 -> Degree/1
  Force 1/1 -> Trigonometric Function1/1
  Force 2/1 -> Trigonometric Function1/2

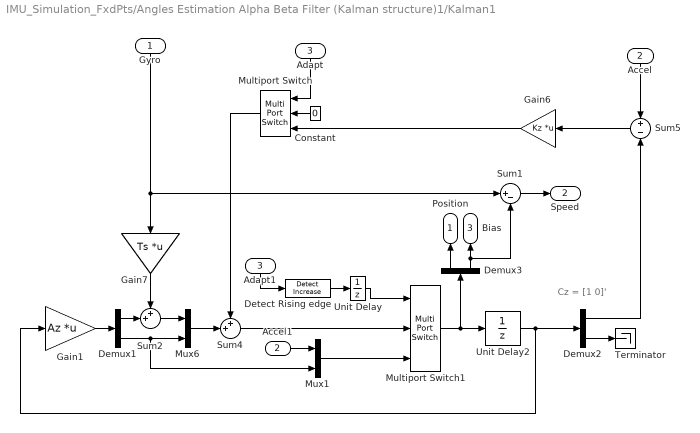
== system IMU_Simulation_FxdPts/Angles Estimation Alpha Beta Filter (Kalman structure)1/Kalman1 ==
  note: Cz = [1 0]'
  Gyro : Inport
  Accel : Inport  Port=2
  Adapt : Inport  Port=3
  Accel1 : InportShadow  Port=2
  Adapt1 : InportShadow  Port=3
  Constant : Constant  Value=0
  Demux1 : Demux  Outputs=2
  Demux2 : Demux  Outputs=2
  Demux3 : Demux  Outputs=2
  Detect Rising edge : simulink/Logic and Bit Operations/Detect Increase  vinit=0  InputProcessing=Inherited  OutDataTypeStr=uint8
  Gain1 : Gain  Gain=Az  Multiplication=Matrix(K*u)
  Gain6 : Gain  Gain=Kz  Multiplication=Matrix(K*u)
  Gain7 : Gain  Gain=Ts  Multiplication=Matrix(K*u)
  Multiport Switch : MultiPortSwitch  DataPortOrder=Zero-based contiguous  Inputs=2  zeroidx=on
  Multiport Switch1 : MultiPortSwitch  DataPortOrder=Zero-based contiguous  Inputs=2  zeroidx=on
  Mux1 : Mux  Inputs=2
  Mux6 : Mux  Inputs=2
  Sum1 : Sum  Inputs=|+-
  Sum2 : Sum  Inputs=++|
  Sum4 : Sum  Inputs=++|
  Sum5 : Sum  Inputs=+-
  Terminator : Terminator
  Unit Delay : UnitDelay  SampleTime=-1
  Unit Delay2 : UnitDelay  SampleTime=-1
  Position : Outport
  Speed : Outport  Port=2
  Bias : Outport  Port=3
  wires:
  Demux2/2 -> Terminator/1
  Mux1/1 -> Multiport Switch1/3
  Accel1/1 -> Mux1/1
  Adapt1/1 -> Detect Rising edge/1
  Sum4/1 -> Multiport Switch1/2
  Multiport Switch1/1 -> Unit Delay2/1, Demux3/1
  Detect Rising edge/1 -> Unit Delay/1
  Constant/1 -> Multiport Switch/2
  Gain6/1 -> Multiport Switch/3
  Adapt/1 -> Multiport Switch/1
  Multiport Switch/1 -> Sum4/1
  Demux2/1 -> Sum5/2
  Gain1/1 -> Demux1/1
  Demux1/1 -> Sum2/2
  Sum2/1 -> Mux6/1
  Demux1/2 -> Mux1/2, Mux6/2
  Mux6/1 -> Sum4/2
  Sum5/1 -> Gain6/1
  Gain7/1 -> Sum2/1
  Accel/1 -> Sum5/1
  Gyro/1 -> Gain7/1, Sum1/1
  Unit Delay/1 -> Multiport Switch1/1
  Unit Delay2/1 -> Demux2/1, Gain1/1
  Demux3/1 -> Position/1
  Demux3/2 -> Bias/1, Sum1/2
  Sum1/1 -> Speed/1

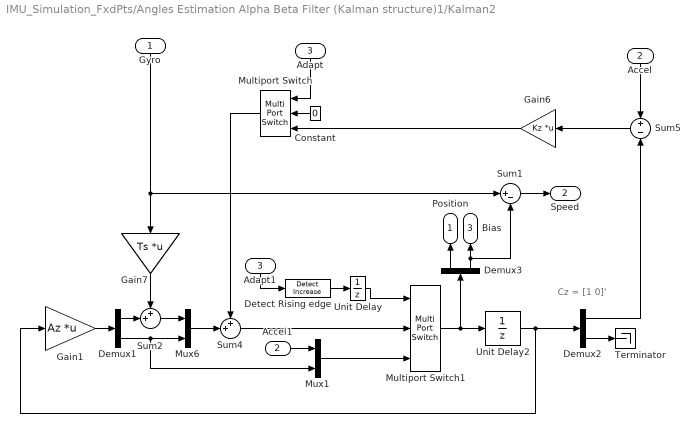
== system IMU_Simulation_FxdPts/Angles Estimation Alpha Beta Filter (Kalman structure)1/Kalman2 ==
  note: Cz = [1 0]'
  Gyro : Inport
  Accel : Inport  Port=2
  Adapt : Inport  Port=3
  Accel1 : InportShadow  Port=2
  Adapt1 : InportShadow  Port=3
  Constant : Constant  Value=0
  Demux1 : Demux  Outputs=2
  Demux2 : Demux  Outputs=2
  Demux3 : Demux  Outputs=2
  Detect Rising edge : simulink/Logic and Bit Operations/Detect Increase  vinit=0  InputProcessing=Inherited  OutDataTypeStr=uint8
  Gain1 : Gain  Gain=Az  Multiplication=Matrix(K*u)
  Gain6 : Gain  Gain=Kz  Multiplication=Matrix(K*u)
  Gain7 : Gain  Gain=Ts  Multiplication=Matrix(K*u)
  Multiport Switch : MultiPortSwitch  DataPortOrder=Zero-based contiguous  Inputs=2  zeroidx=on
  Multiport Switch1 : MultiPortSwitch  DataPortOrder=Zero-based contiguous  Inputs=2  zeroidx=on
  Mux1 : Mux  Inputs=2
  Mux6 : Mux  Inputs=2
  Sum1 : Sum  Inputs=|+-
  Sum2 : Sum  Inputs=++|
  Sum4 : Sum  Inputs=++|  OutDataTypeStr=Inherit: Inherit via back propagation
  Sum5 : Sum  Inputs=+-
  Terminator : Terminator
  Unit Delay : UnitDelay  SampleTime=-1
  Unit Delay2 : UnitDelay  SampleTime=-1
  Position : Outport
  Speed : Outport  Port=2
  Bias : Outport  Port=3
  wires:
  Sum1/1 -> Speed/1
  Demux3/2 -> Sum1/2, Bias/1
  Demux3/1 -> Position/1
  Unit Delay2/1 -> Gain1/1, Demux2/1
  Unit Delay/1 -> Multiport Switch1/1
  Gyro/1 -> Sum1/1, Gain7/1
  Accel/1 -> Sum5/1
  Gain7/1 -> Sum2/1
  Sum5/1 -> Gain6/1
  Mux6/1 -> Sum4/2
  Demux1/2 -> Mux6/2, Mux1/2
  Sum2/1 -> Mux6/1
  Demux1/1 -> Sum2/2
  Gain1/1 -> Demux1/1
  Demux2/1 -> Sum5/2
  Multiport Switch/1 -> Sum4/1
  Adapt/1 -> Multiport Switch/1
  Gain6/1 -> Multiport Switch/3
  Constant/1 -> Multiport Switch/2
  Detect Rising edge/1 -> Unit Delay/1
  Multiport Switch1/1 -> Demux3/1, Unit Delay2/1
  Sum4/1 -> Multiport Switch1/2
  Adapt1/1 -> Detect Rising edge/1
  Accel1/1 -> Mux1/1
  Mux1/1 -> Multiport Switch1/3
  Demux2/2 -> Terminator/1

== system IMU_Simulation_FxdPts/Angles Estimation Alpha Beta Filter (Kalman structure)1/Norm L1 ==
  Accel Y : Inport
  Accel Z : Inport  Port=2
  Accel X : Inport  Port=3
  Abs : Abs
  Abs1 : Abs
  Abs2 : Abs
  Sum1 : Sum
  Sum3 : Sum
  abs(Y)+abs(Z) : Outport
  abs(X)+abs(Z) : Outport  Port=2
  wires:
  Sum1/1 -> abs(X)+abs(Z)/1
  Accel X/1 -> Abs2/1
  Abs2/1 -> Sum1/2
  Sum3/1 -> abs(Y)+abs(Z)/1
  Accel Z/1 -> Abs1/1
  Accel Y/1 -> Abs/1
  Abs1/1 -> Sum3/2, Sum1/1
  Abs/1 -> Sum3/1

== system IMU_Simulation_FxdPts/Angles Estimation Alpha Beta Filter (Kalman structure)1/Simplified Kalman for publi ==
  note: Cz = [1 0]'
  Gyro : Inport
  Accel : Inport  Port=2
  Demux1 : Demux  Outputs=2
  Demux2 : Demux  Outputs=2
  Gain1 : Gain  Gain=Az  Multiplication=Matrix(K*u)
  Gain6 : Gain  Gain=Kz  Multiplication=Matrix(K*u)
  Gain7 : Gain  Gain=Ts  Multiplication=Matrix(K*u)
  Mux6 : Mux  Inputs=2
  Sum2 : Sum  Inputs=++|
  Sum4 : Sum  Inputs=++|
  Sum5 : Sum  Inputs=+-
  Terminator : Terminator
  Unit Delay2 : UnitDelay  SampleTime=-1
  Angle Estimation : Outport
  wires:
  Gain6/1 -> Sum4/1
  Unit Delay2/1 -> Gain1/1, Demux2/1
  Gyro/1 -> Gain7/1
  Accel/1 -> Sum5/1
  Gain7/1 -> Sum2/1
  Sum5/1 -> Gain6/1
  Mux6/1 -> Sum4/2
  Demux1/2 -> Mux6/2  "Gyro Bias"
  Sum2/1 -> Mux6/1  "Angle Estimation"
  Demux1/1 -> Sum2/2
  Gain1/1 -> Demux1/1
  Demux2/1 -> Angle Estimation/1, Sum5/2
  Sum4/1 -> Unit Delay2/1
  Demux2/2 -> Terminator/1

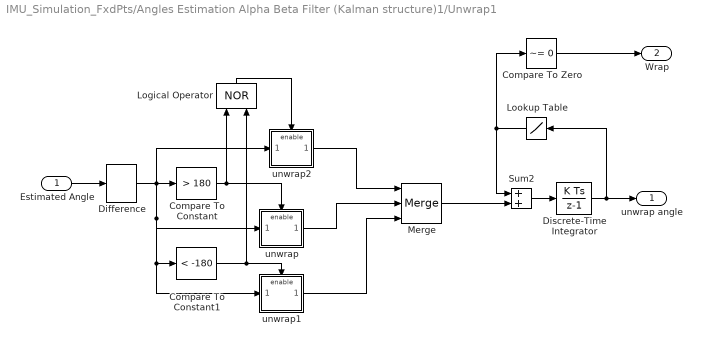
== system IMU_Simulation_FxdPts/Angles Estimation Alpha Beta Filter (Kalman structure)1/Unwrap1 ==
  Estimated Angle : Inport
  Compare To Constant : simulink/Logic and Bit Operations/Compare To Constant  relop=>  const=180  OutDataTypeStr=uint8  ZeroCross=off
  Compare To Constant1 : simulink/Logic and Bit Operations/Compare To Constant  relop=<  const=-180  OutDataTypeStr=uint8  ZeroCross=off
  Compare To Zero : simulink/Logic and Bit Operations/Compare To Zero  relop=~=  OutDataTypeStr=uint8  ZeroCross=off
  Difference : simulink/Discrete/Difference  ICPrevInput=0.0  InputProcessing=Inherited  OutMin=[]  OutMax=[]  OutDataType=sfix(16)  OutScaling=2^-10  DoSatur=off
  Discrete-Time Integrator : DiscreteIntegrator  gainval=1000  SampleTime=-1  ICPrevOutput=DiscIntNeverNeededParam  ICPrevScaledInput=DiscIntNeverNeededParam
  Logical Operator : Logic  Operator=NOR  AllPortsSameDT=off  OutDataTypeStr=boolean
  Lookup Table : Lookup  InputValues=[-500 -195 195]  Table=[+360 0 -360]  LookUpMeth=Use Input Below
  Merge : Merge  Inputs=3
  Sum2 : Sum
  unwrap : Subsystem  TreatAsAtomicUnit=on
  unwrap1 : Subsystem  TreatAsAtomicUnit=on
  unwrap2 : Subsystem  TreatAsAtomicUnit=on
  unwrap angle : Outport
  Wrap : Outport  Port=2
  wires:
  Discrete-Time Integrator/1 -> unwrap angle/1, Lookup Table/1
  Estimated Angle/1 -> Difference/1
  unwrap1/1(Out1) -> Merge/3
  unwrap/1(Out1) -> Merge/2
  unwrap2/1(Out1) -> Merge/1
  Logical Operator/1 -> unwrap2/Enable
  Compare To Constant1/1 -> Logical Operator/2, unwrap1/Enable
  Compare To Constant/1 -> unwrap/Enable, Logical Operator/1
  Difference/1 -> unwrap2/1(In1), unwrap1/1(In1), Compare To Constant1/1, unwrap/1(In1), Compare To Constant/1
  Sum2/1 -> Discrete-Time Integrator/1
  Merge/1 -> Sum2/2
  Lookup Table/1 -> Sum2/1, Compare To Zero/1
  Compare To Zero/1 -> Wrap/1

== system IMU_Simulation_FxdPts/Angles Estimation Alpha Beta Filter (Kalman structure)1/Unwrap2 ==
  Estimated Angle : Inport
  Compare To Constant : simulink/Logic and Bit Operations/Compare To Constant  relop=>  const=180  OutDataTypeStr=uint8  ZeroCross=off
  Compare To Constant1 : simulink/Logic and Bit Operations/Compare To Constant  relop=<  const=-180  OutDataTypeStr=uint8  ZeroCross=off
  Compare To Zero : simulink/Logic and Bit Operations/Compare To Zero  relop=~=  OutDataTypeStr=uint8  ZeroCross=off
  Difference : simulink/Discrete/Difference  ICPrevInput=0.0  InputProcessing=Inherited  OutMin=[]  OutMax=[]  OutDataType=sfix(16)  OutScaling=2^-10  DoSatur=off
  Discrete-Time Integrator : DiscreteIntegrator  gainval=1000  SampleTime=-1  ICPrevOutput=DiscIntNeverNeededParam  ICPrevScaledInput=DiscIntNeverNeededParam
  Logical Operator : Logic  Operator=NOR  AllPortsSameDT=off  OutDataTypeStr=boolean
  Lookup Table : Lookup  InputValues=[-500 -195 195]  Table=[+360 0 -360]  LookUpMeth=Use Input Below
  Merge : Merge  Inputs=3
  Sum2 : Sum
  unwrap : Subsystem  TreatAsAtomicUnit=on
  unwrap1 : Subsystem  TreatAsAtomicUnit=on
  unwrap2 : Subsystem  TreatAsAtomicUnit=on
  unwrap angle : Outport
  Wrap : Outport  Port=2
  wires:
  Compare To Zero/1 -> Wrap/1
  Lookup Table/1 -> Compare To Zero/1, Sum2/1
  Merge/1 -> Sum2/2
  Sum2/1 -> Discrete-Time Integrator/1
  Difference/1 -> Compare To Constant/1, unwrap/1(In1), Compare To Constant1/1, unwrap1/1(In1), unwrap2/1(In1)
  Compare To Constant/1 -> Logical Operator/1, unwrap/Enable
  Compare To Constant1/1 -> unwrap1/Enable, Logical Operator/2
  Logical Operator/1 -> unwrap2/Enable
  unwrap2/1(Out1) -> Merge/1
  unwrap/1(Out1) -> Merge/2
  unwrap1/1(Out1) -> Merge/3
  Estimated Angle/1 -> Difference/1
  Discrete-Time Integrator/1 -> Lookup Table/1, unwrap angle/1

== system IMU_Simulation_FxdPts/Angles Estimation Alpha Beta Filter (Kalman structure) Fxt Points1/Unwrap1/unwrap ==
  In1 : Inport
  Enable : EnablePort
  Bias2 : Constant  Value=-360  OutDataTypeStr=Inherit: Inherit via back propagation
  Sum2 : Sum  OutDataTypeStr=Inherit: Same as first input
  Out1 : Outport
  wires:
  Bias2/1 -> Sum2/2
  Sum2/1 -> Out1/1
  In1/1 -> Sum2/1

== system IMU_Simulation_FxdPts/Angles Estimation Alpha Beta Filter (Kalman structure) Fxt Points1/Unwrap1/unwrap1 ==
  In1 : Inport
  Enable : EnablePort
  Bias2 : Constant  Value=360  OutDataTypeStr=Inherit: Inherit via back propagation
  Sum2 : Sum  OutDataTypeStr=Inherit: Same as first input
  Out1 : Outport
  wires:
  Sum2/1 -> Out1/1
  Bias2/1 -> Sum2/2
  In1/1 -> Sum2/1

== system IMU_Simulation_FxdPts/Angles Estimation Alpha Beta Filter (Kalman structure) Fxt Points1/Unwrap1/unwrap2 ==
  In1 : Inport
  Enable : EnablePort
  Out1 : Outport
  wires:
  In1/1 -> Out1/1

== system IMU_Simulation_FxdPts/Angles Estimation Alpha Beta Filter (Kalman structure) Fxt Points1/Unwrap2/unwrap ==
  In1 : Inport
  Enable : EnablePort
  Bias2 : Constant  Value=-360  OutDataTypeStr=Inherit: Inherit via back propagation
  Sum2 : Sum  OutDataTypeStr=Inherit: Same as first input
  Out1 : Outport
  wires:
  In1/1 -> Sum2/1
  Sum2/1 -> Out1/1
  Bias2/1 -> Sum2/2

== system IMU_Simulation_FxdPts/Angles Estimation Alpha Beta Filter (Kalman structure) Fxt Points1/Unwrap2/unwrap1 ==
  In1 : Inport
  Enable : EnablePort
  Bias2 : Constant  Value=360  OutDataTypeStr=Inherit: Inherit via back propagation
  Sum2 : Sum  OutDataTypeStr=Inherit: Same as first input
  Out1 : Outport
  wires:
  In1/1 -> Sum2/1
  Bias2/1 -> Sum2/2
  Sum2/1 -> Out1/1

== system IMU_Simulation_FxdPts/Angles Estimation Alpha Beta Filter (Kalman structure) Fxt Points1/Unwrap2/unwrap2 ==
  In1 : Inport
  Enable : EnablePort
  Out1 : Outport
  wires:
  In1/1 -> Out1/1

== system IMU_Simulation_FxdPts/Angles Estimation Alpha Beta Filter (Kalman structure)1/Unwrap1/unwrap ==
  In1 : Inport
  Enable : EnablePort
  Bias2 : Constant  Value=-360
  Sum2 : Sum
  Out1 : Outport
  wires:
  Bias2/1 -> Sum2/2
  Sum2/1 -> Out1/1
  In1/1 -> Sum2/1

== system IMU_Simulation_FxdPts/Angles Estimation Alpha Beta Filter (Kalman structure)1/Unwrap1/unwrap1 ==
  In1 : Inport
  Enable : EnablePort
  Bias2 : Constant  Value=360
  Sum2 : Sum
  Out1 : Outport
  wires:
  Sum2/1 -> Out1/1
  Bias2/1 -> Sum2/2
  In1/1 -> Sum2/1

== system IMU_Simulation_FxdPts/Angles Estimation Alpha Beta Filter (Kalman structure)1/Unwrap1/unwrap2 ==
  In1 : Inport
  Enable : EnablePort
  Out1 : Outport
  wires:
  In1/1 -> Out1/1

== system IMU_Simulation_FxdPts/Angles Estimation Alpha Beta Filter (Kalman structure)1/Unwrap2/unwrap ==
  In1 : Inport
  Enable : EnablePort
  Bias2 : Constant  Value=-360
  Sum2 : Sum
  Out1 : Outport
  wires:
  In1/1 -> Sum2/1
  Sum2/1 -> Out1/1
  Bias2/1 -> Sum2/2

== system IMU_Simulation_FxdPts/Angles Estimation Alpha Beta Filter (Kalman structure)1/Unwrap2/unwrap1 ==
  In1 : Inport
  Enable : EnablePort
  Bias2 : Constant  Value=360
  Sum2 : Sum
  Out1 : Outport
  wires:
  In1/1 -> Sum2/1
  Bias2/1 -> Sum2/2
  Sum2/1 -> Out1/1

== system IMU_Simulation_FxdPts/Angles Estimation Alpha Beta Filter (Kalman structure)1/Unwrap2/unwrap2 ==
  In1 : Inport
  Enable : EnablePort
  Out1 : Outport
  wires:
  In1/1 -> Out1/1
